simulink model "tp290284"  (Simulink 3.0)
settings: Solver=ode1  SolverMode=SingleTasking  StartTime=0.0  StopTime=35  FixedStep=Ts  RelTol=1e-3
values from neighbouring files (symbols this model uses):
  K = input('Put open loop gain K = (15) ')    [init_I0_disc2.m]    (also in init_PI0_windupless.m = input('Put identified integrator gain value K (8) = '); step_resp1.mat = 15)
  Tfil = 4*Ta    [init_I0_disc2.m]    (also in init_PI0_windupless.m = 4*(T1+Ts); init_PI1_windupless.m = 4.337*Td; step_resp1.mat = 1.2)
  Ts = 0.2    [init_I0_disc2.m]    (also in init_PI0_windupless.m = 0.5; init_PI1_windupless.m; init_PID.m; step_resp1.mat)
  Umax = 5    [init_I0_disc2.m]    (also in init_PI0_windupless.m; init_PI1_windupless.m; init_PID.m; step_resp1.mat)
  Umin = 0    [init_I0_disc2.m]    (also in init_PI0_windupless.m; init_PI1_windupless.m; init_PID.m; step_resp1.mat)
libraries: simulink x1, udaq28LT_lib x1
settings Model: LastModifiedBy=mato  ExtModeMexFile=rtwinext  ExtModeTrigDuration=100000  SaveFormat=Matrix  RTWSystemTargetFile=rtwin.tlc  RTWTemplateMakefile=rtwintmf  RTWOptions="-aCCOptimize=1 -aEnforceIntegerDowncast=1 -aExtMode=1 -aFoldNonRolledExpr=1 -aForceParamTrailComments=0 -aGenerateComments=1 -aGenerateReport=0 -aIncDataTypeInIds=0 -aIncHierarchyInIds=0 -aInlineInvariantSignals=0 -aInlinedPrmAccess=\"Literals\" -aLocalBlockOutputs=1 -aMaxRTWIdLen=31 -aPrefixModelToSubsysFcnNames=1 -aRTWVerbose=1 -aRebuildAll=1 -aRollThreshold=5 -aShowEliminatedStatements=1"

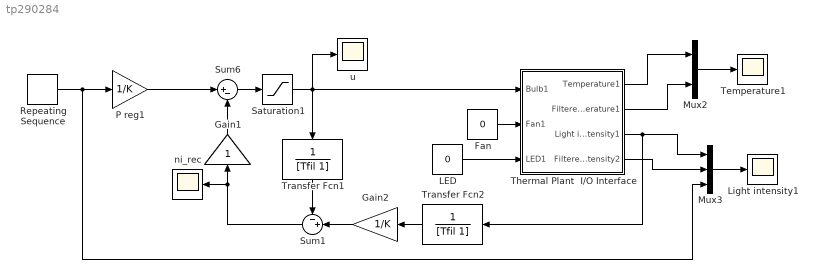
== system tp290284 ==
  Fan : Constant  Value=0
  Gain1 : Gain  Orientation=up  Gain=1  SaturateOnIntegerOverflow=on
  Gain2 : Gain  Orientation=left  Gain=1/K  SaturateOnIntegerOverflow=on
  LED : Constant  Value=0
  Light intensity1 : Scope
      settings: TickLabels=on  TimeRange=30  YMin=0  YMax=100  SaveName=yl  DataFormat=Matrix
  Mux2 : Mux  Inputs=2
  Mux3 : Mux  Inputs=3
  P reg1 : Gain  Gain=1/K  SaturateOnIntegerOverflow=on
  Repeating Sequence : simulink/Sources/Repeating Sequence  rep_seq_t="[0  7 7 14 14 21 21 28 28 35]"  rep_seq_y=[20 20 30 30 25 25 15 15 40 40]
  Saturation1 : Saturate  UpperLimit=Umax  LowerLimit=Umin
  Sum1 : Sum  Orientation=left  Inputs=-+|  SaturateOnIntegerOverflow=on
  Sum6 : Sum  Inputs=|+-  SaturateOnIntegerOverflow=on
  Temperature1 : Scope
      settings: TickLabels=on  TimeRange=30  YMin=15  YMax=50  SaveName=yt  DataFormat=Matrix
  Thermal Plant  I/O Interface : Subsystem
      mask Display: disp('Thermo-optical\nPlant\nI/O Interface')
  Transfer Fcn1 : TransferFcn  Orientation=down  Numerator=[1]  Denominator=[Tfil 1]
  Transfer Fcn2 : TransferFcn  Orientation=left  Numerator=[1]  Denominator=[Tfil 1]
  ni_rec : Scope
      settings: TimeRange=auto  YMin=1.5  YMax=2.7  SaveName=ni_rec  DataFormat=Matrix  Decimation=10  SampleInput=on  SampleTime=Ts
  u : Scope
      settings: TimeRange=40  YMin=-0.5  YMax=5.5  SaveName=u  DataFormat=Matrix  Decimation=10  SampleInput=on  SampleTime=Ts
  wires:
  Sum6/1 -> Saturation1/1
  P reg1/1 -> Sum6/1
  Transfer Fcn1/1 -> Sum1/1
  Sum1/1 -> ni_rec/1, Gain1/1
  Saturation1/1 -> u/1, Transfer Fcn1/1, Thermal Plant  I/O Interface/1(Bulb1)
  Gain1/1 -> Sum6/2
  Transfer Fcn2/1 -> Gain2/1
  Gain2/1 -> Sum1/2
  Repeating Sequence/1 -> P reg1/1, Mux3/3
  Mux2/1 -> Temperature1/1
  Mux3/1 -> Light intensity1/1
  Fan/1 -> Thermal Plant  I/O Interface/2(Fan1)
  LED/1 -> Thermal Plant  I/O Interface/3(LED1)
  Thermal Plant  I/O Interface/1(Temperature1) -> Mux2/1
  Thermal Plant  I/O Interface/2(Filtered  temperature1) -> Mux2/2
  Thermal Plant  I/O Interface/3(Light intensity1) -> Mux3/1, Transfer Fcn2/1
  Thermal Plant  I/O Interface/4(Filtered  light intensity2) -> Mux3/2

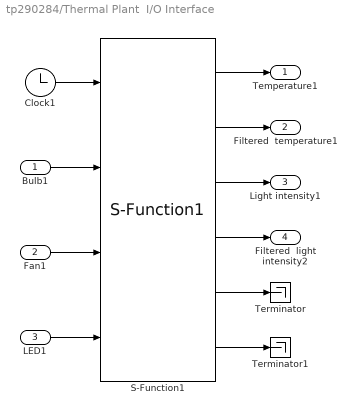
== system tp290284/Thermal Plant  I/O Interface ==
  Bulb1 : Inport  Port=1  PortWidth=-1  SampleTime=-1  DataType=auto
      settings: SignalType=auto
  Fan1 : Inport  Port=2  PortWidth=-1  SampleTime=-1  DataType=auto
      settings: SignalType=auto
  LED1 : Inport  Port=3  PortWidth=-1  SampleTime=-1  DataType=auto
      settings: SignalType=auto
  Clock1 : Clock
      settings: DisplayTime=off  Decimation=10
  S-Function1 : udaq28LT_lib/S-Function1  Priority=1  com_port=COM3  Ts=Ts  events_ot=2  rd_timeout=Ts/2*1000  matlab_prior=ABOVE_NORMAL_PRIORITY  warning=on  printout=off
  Terminator : Terminator
  Terminator1 : Terminator
  Temperature1 : Outport  Port=1
  Filtered  temperature1 : Outport  Port=2
  Light intensity1 : Outport  Port=3
  Filtered  light intensity2 : Outport  Port=4
  wires:
  S-Function1/1 -> Temperature1/1
  S-Function1/2 -> Filtered  temperature1/1
  Clock1/1 -> S-Function1/1
  Bulb1/1 -> S-Function1/2
  Fan1/1 -> S-Function1/3
  S-Function1/3 -> Light intensity1/1
  S-Function1/4 -> Filtered  light intensity2/1
  S-Function1/5 -> Terminator/1
  S-Function1/6 -> Terminator1/1
  LED1/1 -> S-Function1/4
